simulink model "KR6_CLIK"  (R2018a)
settings: Solver=VariableStepAuto  StartTime=0.0  StopTime=inf  RelTol=1e-3
libraries: vrlib x8, KR6_Lib x1, realtime_pacer_lib x1
settings Model: Creator=Pedro Ramalho  LastModifiedBy=Pedro Ramalho

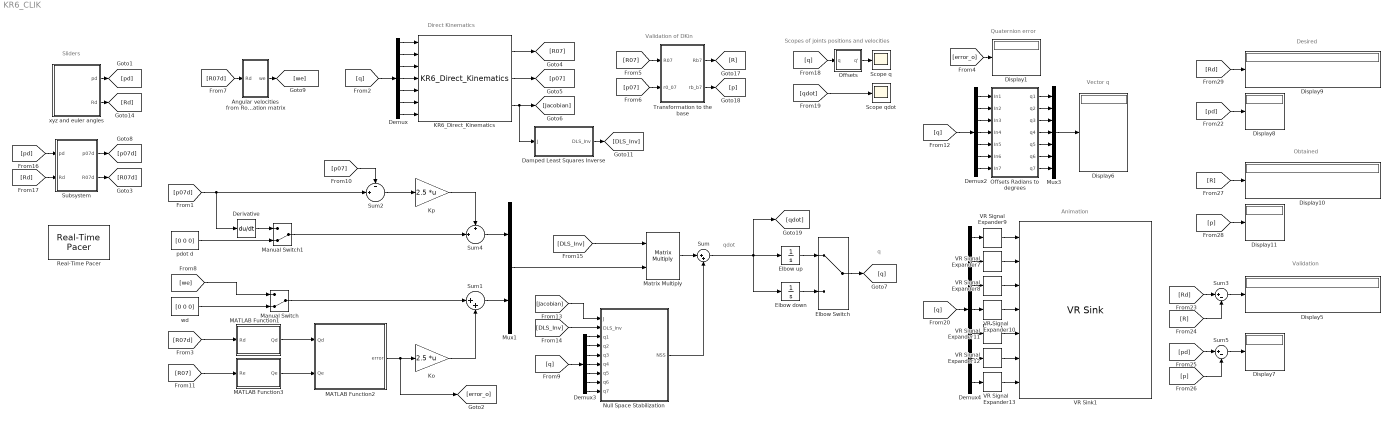
== system KR6_CLIK ==
  note: Direct Kinematics
  note: Validation of DKin
  note: qdot
  note: q
  note: Sliders
  note: Desired
  note: Obtained
  note: Validation
  note: Vector q
  note: Animation
  note: Scopes of joints positions and velocities
  note: Quaternion error
  Angular velocities from Rotation matrix : Subsystem
  Damped Least Squares Inverse : MATLAB Function  TreatAsAtomicUnit=on
  Demux{,2..4} (4 alike) : Demux  Outputs=7
  Derivative : Derivative
  Display{1,5..11} (8 alike) : Display
  Elbow Switch : ManualSwitch
  Elbow down : Integrator  InitialCondition=[0 0 0 -pi/2 0 0 pi]  ZeroCross=off
  Elbow up : Integrator  InitialCondition=[0 pi/8 -pi/2 0 0 0 pi]  ZeroCross=off
  KR6_Direct_Kinematics : KR6_Lib/KR6_Direct_Kinematics
  Ko : Gain  Gain=2.5  Multiplication=Matrix(K*u)
  Kp : Gain  Gain=2.5  Multiplication=Matrix(K*u)
  MATLAB Function1 : MATLAB Function  TreatAsAtomicUnit=on
  MATLAB Function2 : MATLAB Function  TreatAsAtomicUnit=on
  MATLAB Function3 : MATLAB Function  TreatAsAtomicUnit=on
  Manual Switch : ManualSwitch  CurrentSetting=0
  Manual Switch1 : ManualSwitch  CurrentSetting=0
  Matrix Multiply : Product  Multiplication=Matrix(*)
  Mux1 : Mux  Inputs=2
  Mux3 : Mux  Inputs=7
  Null Space Stabilization : MATLAB Function  TreatAsAtomicUnit=on
  Offsets : Subsystem
  Offsets Radians to degrees : Subsystem
  Real-Time Pacer : realtime_pacer_lib/Real-Time Pacer  simTimePerRealTime=1
  Scope q : Scope
  Scope qdot : Scope
  Subsystem : Subsystem
  Sum : Sum  Inputs=|++
  Sum1 : Sum  Inputs=|++
  Sum2 : Sum  Inputs=-|+||
  Sum3 : Sum  Inputs=|+-
  Sum4 : Sum  Inputs=+|+||
  Sum5 : Sum  Inputs=|+-
  Transformation to the base : Subsystem
  VR Signal Expander{7..8,10..13} (6 alike) : vrlib/VR Signal Expander  outwidth=4  outidx=4
      settings: SourceProductName=Simulink 3D Animation  SourceProductBaseCode=VR
  VR Signal Expander9 : vrlib/VR Signal Expander  outwidth=3  outidx=3
      settings: SourceProductName=Simulink 3D Animation  SourceProductBaseCode=VR
  VR Sink1 : vrlib/VR Sink  InstantiateOnLoad=on  SampleTime=0.1  ViewEnable=on  RemoteChange=off  RemoteView=off  FieldsWritten=Jt1_DH_dv.translation.3.1.1.double#Jt2_DH_dv.rotation.4.1.1.double#Jt3_DH_dv.rotation.4.1.1.double#Jt4_DH_dv.rotation.4.1.1.double#Jt5_DH_dv.rotation.4.1.1.double#Jt6_DH_dv.rotation.4.1.1.double#Jt7_DH_dv.rotation.4.1.1.double  WorldFileName=vrrobotKR6.wrl  WorldDescription=D-H Reference Frames for Virtual Reality Robot  AutoView=off  VideoDimensions=[]  AllowVariableSize=off
      settings: SourceProductBaseCode=VR
  pdot d : Constant  Value=[0 0 0]
  wd : Constant  Value=[0 0 0]
  xyz and euler angles : Subsystem  mask{px=0.20163, py=0.44482, pz=0.97382, phi=-75.4157, theta=-8.5121, psi=-120.3774}
      mask prompts: px "x"; py "y"; pz "z"
      mask DialogControl ParameterGroupVar_copy Prompt: Euler angles
  wires:
  KR6_Direct_Kinematics/1 -> [R07]
  KR6_Direct_Kinematics/2 -> [p07]
  KR6_Direct_Kinematics/3 -> [Jacobian], Damped Least Squares Inverse/1(J)
  Demux/1 -> KR6_Direct_Kinematics/1
  Demux/2 -> KR6_Direct_Kinematics/2
  Demux/3 -> KR6_Direct_Kinematics/3
  Demux/4 -> KR6_Direct_Kinematics/4
  Demux/5 -> KR6_Direct_Kinematics/5
  Demux/6 -> KR6_Direct_Kinematics/6
  Demux/7 -> KR6_Direct_Kinematics/7
  [q] -> Demux/1
  [p07d] -> Sum2/2, Derivative/1
  Transformation to the base/2(rb_b7) -> [p]
  [R07] -> Transformation to the base/1(R07)
  [p07] -> Transformation to the base/2(r0_07)
  [R07d] -> MATLAB Function1/1(Rd)
  MATLAB Function1/1(Qd) -> MATLAB Function2/1(Qd)
  MATLAB Function2/1(error) -> [error_o], Ko/1
  Ko/1 -> Sum1/2
  wd/1 -> Manual Switch/2
  Derivative/1 -> Manual Switch1/1
  pdot d/1 -> Manual Switch1/2
  [R07d] -> Angular velocities from Rotation matrix/1(Rd)
  Angular velocities from Rotation matrix/1(we) -> [we]
  [we] -> Manual Switch/1
  Manual Switch1/1 -> Sum4/2
  Kp/1 -> Sum4/1
  Manual Switch/1 -> Sum1/1
  Sum4/1 -> Mux1/1
  Sum1/1 -> Mux1/2
  Elbow up/1 -> Elbow Switch/1
  [p07] -> Sum2/1
  [R07] -> MATLAB Function3/1(Re)
  MATLAB Function3/1(Qe) -> MATLAB Function2/2(Qe)
  Offsets Radians to degrees/5(q5) -> Mux3/5
  Demux2/4 -> Offsets Radians to degrees/4(In4)
  Offsets Radians to degrees/3(q3) -> Mux3/3
  [q] -> Demux2/1
  Demux2/3 -> Offsets Radians to degrees/3(In3)
  Offsets Radians to degrees/1(q1) -> Mux3/1
  Demux2/6 -> Offsets Radians to degrees/6(In6)
  Demux2/5 -> Offsets Radians to degrees/5(In5)
  Offsets Radians to degrees/7(q7) -> Mux3/7
  Offsets Radians to degrees/4(q4) -> Mux3/4
  Mux3/1 -> Display6/1
  Offsets Radians to degrees/2(q2) -> Mux3/2
  Demux2/2 -> Offsets Radians to degrees/2(In2)
  Demux2/1 -> Offsets Radians to degrees/1(In1)
  Offsets Radians to degrees/6(q6) -> Mux3/6
  Demux2/7 -> Offsets Radians to degrees/7(In7)
  Damped Least Squares Inverse/1(DLS_Inv) -> [DLS_Inv]
  Matrix Multiply/1 -> Sum/1
  Null Space Stabilization/1(NSS) -> Sum/2
  Mux1/1 -> Matrix Multiply/2
  [q] -> Demux3/1
  Demux3/5 -> Null Space Stabilization/7(q5)
  Demux3/7 -> Null Space Stabilization/9(q7)
  Demux3/2 -> Null Space Stabilization/4(q2)
  Demux3/1 -> Null Space Stabilization/3(q1)
  Demux3/3 -> Null Space Stabilization/5(q3)
  Demux3/4 -> Null Space Stabilization/6(q4)
  Demux3/6 -> Null Space Stabilization/8(q6)
  [Jacobian] -> Null Space Stabilization/1(J)
  [DLS_Inv] -> Null Space Stabilization/2(DLS_Inv)
  [DLS_Inv] -> Matrix Multiply/1
  xyz and euler angles/2(Rd) -> [Rd]
  [pd] -> Subsystem/1(pd)
  [Rd] -> Subsystem/2(Rd)
  Subsystem/1(p07d) -> [p07d]
  xyz and euler angles/1(pd) -> [pd]
  Subsystem/2(R07d) -> [R07d]
  Sum5/1 -> Display7/1
  [Rd] -> Display9/1
  [R] -> Sum3/2
  Sum3/1 -> Display5/1
  [p] -> Sum5/2
  [Rd] -> Sum3/1
  [pd] -> Sum5/1
  [p] -> Display11/1
  [pd] -> Display8/1
  [R] -> Display10/1
  Offsets/1(q') -> Scope q/1
  [q] -> Offsets/1(q)
  Sum/1 -> Elbow down/1, Elbow up/1, [qdot]
  Elbow down/1 -> Elbow Switch/2
  Elbow Switch/1 -> [q]
  Sum2/1 -> Kp/1
  Transformation to the base/1(Rb7) -> [R]
  [qdot] -> Scope qdot/1
  Demux4/7 -> VR Signal Expander13/1
  Demux4/4 -> VR Signal Expander10/1
  Demux4/2 -> VR Signal Expander7/1
  Demux4/6 -> VR Signal Expander12/1
  Demux4/1 -> VR Signal Expander9/1
  [q] -> Demux4/1
  VR Signal Expander11/1 -> VR Sink1/5
  VR Signal Expander12/1 -> VR Sink1/6
  VR Signal Expander9/1 -> VR Sink1/1
  VR Signal Expander8/1 -> VR Sink1/3
  VR Signal Expander10/1 -> VR Sink1/4
  Demux4/5 -> VR Signal Expander11/1
  VR Signal Expander13/1 -> VR Sink1/7
  VR Signal Expander7/1 -> VR Sink1/2
  Demux4/3 -> VR Signal Expander8/1
  [error_o] -> Display1/1

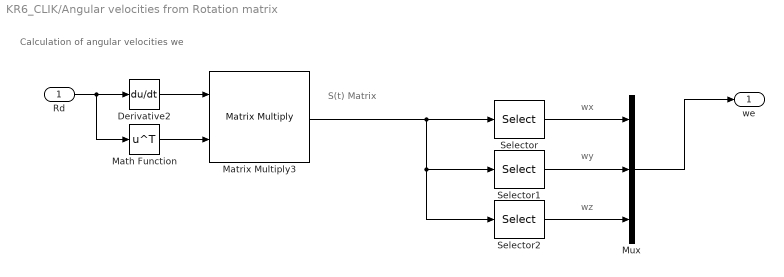
== system KR6_CLIK/Angular velocities from Rotation matrix ==
  note: S(t) Matrix
  note: wx
  note: Calculation of angular velocities we
  note: wz
  note: wy
  Rd : Inport
  Derivative2 : Derivative
  Math Function : Math  Operator=transpose  SaturateOnIntegerOverflow=on
  Matrix Multiply3 : Product  Multiplication=Matrix(*)
  Mux : Mux  Inputs=3
  Selector : Selector  NumberOfDimensions=2  InputPortWidth=3  IndexOptions=Index vector (dialog),Index vector (dialog)  Indices=[3],[2]  OutputSizes=1,1
  Selector1 : Selector  NumberOfDimensions=2  InputPortWidth=3  IndexOptions=Index vector (dialog),Index vector (dialog)  Indices=[1],[3]  OutputSizes=1,1
  Selector2 : Selector  NumberOfDimensions=2  InputPortWidth=3  IndexOptions=Index vector (dialog),Index vector (dialog)  Indices=[2],[1]  OutputSizes=1,1
  we : Outport
  wires:
  Mux/1 -> we/1
  Matrix Multiply3/1 -> Selector2/1, Selector1/1, Selector/1
  Rd/1 -> Math Function/1, Derivative2/1
  Derivative2/1 -> Matrix Multiply3/1
  Math Function/1 -> Matrix Multiply3/2
  Selector1/1 -> Mux/2
  Selector/1 -> Mux/1
  Selector2/1 -> Mux/3

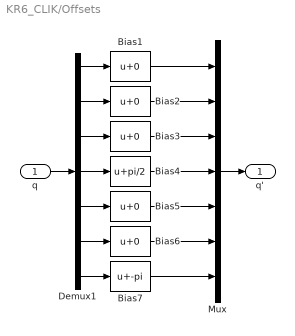
== system KR6_CLIK/Offsets ==
  q : Inport
  Bias{1..3,5..6} (5 alike) : Bias
  Bias4 : Bias  Bias=pi/2
  Bias7 : Bias  Bias=-pi
  Demux1 : Demux  Outputs=7
  Mux : Mux  Inputs=7
  q' : Outport
  wires:
  Bias2/1 -> Mux/2
  Bias3/1 -> Mux/3
  Bias4/1 -> Mux/4
  Bias5/1 -> Mux/5
  Bias6/1 -> Mux/6
  Bias7/1 -> Mux/7
  q/1 -> Demux1/1
  Demux1/1 -> Bias1/1
  Demux1/2 -> Bias2/1
  Demux1/3 -> Bias3/1
  Demux1/4 -> Bias4/1
  Demux1/5 -> Bias5/1
  Demux1/6 -> Bias6/1
  Demux1/7 -> Bias7/1
  Bias1/1 -> Mux/1
  Mux/1 -> q'/1

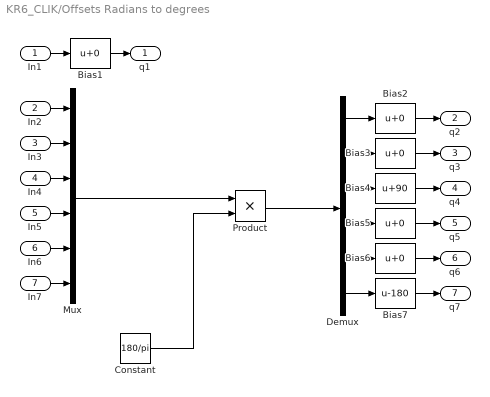
== system KR6_CLIK/Offsets Radians to degrees ==
  In1 : Inport
  In2 : Inport  Port=2
  In3 : Inport  Port=3
  In4 : Inport  Port=4
  In5 : Inport  Port=5
  In6 : Inport  Port=6
  In7 : Inport  Port=7
  Bias{1..3,5..6} (5 alike) : Bias
  Bias4 : Bias  Bias=90
  Bias7 : Bias  Bias=-180
  Constant : Constant  Value=180/pi
  Demux : Demux  Outputs=6
  Mux : Mux  Inputs=6
  Product : Product
  q1 : Outport
  q2 : Outport  Port=2
  q3 : Outport  Port=3
  q4 : Outport  Port=4
  q5 : Outport  Port=5
  q6 : Outport  Port=6
  q7 : Outport  Port=7
  wires:
  In1/1 -> Bias1/1
  Bias1/1 -> q1/1
  Mux/1 -> Product/1
  Constant/1 -> Product/2
  Product/1 -> Demux/1
  In2/1 -> Mux/1
  In3/1 -> Mux/2
  In4/1 -> Mux/3
  In5/1 -> Mux/4
  In6/1 -> Mux/5
  In7/1 -> Mux/6
  Demux/1 -> Bias2/1
  Demux/2 -> Bias3/1
  Demux/3 -> Bias4/1
  Demux/4 -> Bias5/1
  Demux/5 -> Bias6/1
  Demux/6 -> Bias7/1
  Bias2/1 -> q2/1
  Bias3/1 -> q3/1
  Bias4/1 -> q4/1
  Bias5/1 -> q5/1
  Bias6/1 -> q6/1
  Bias7/1 -> q7/1

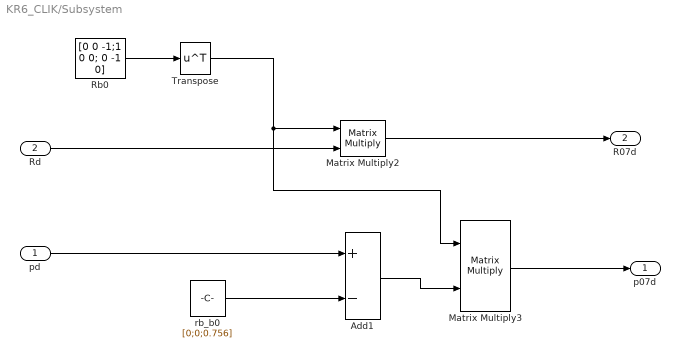
== system KR6_CLIK/Subsystem ==
  pd : Inport
  Rd : Inport  Port=2
  Add1 : Sum  Inputs=+-
  Matrix Multiply2 : Product  Multiplication=Matrix(*)
  Matrix Multiply3 : Product  Multiplication=Matrix(*)
  Rb0 : Constant  Value=[0 0 -1;1 0 0; 0 -1 0]
  Transpose : Math  Operator=transpose  SaturateOnIntegerOverflow=on
  rb_b0 : Constant  Value=[0;0;0.756]
  p07d : Outport
  R07d : Outport  Port=2
  wires:
  Add1/1 -> Matrix Multiply3/2
  Matrix Multiply3/1 -> p07d/1
  Rb0/1 -> Transpose/1
  Transpose/1 -> Matrix Multiply3/1, Matrix Multiply2/1
  Rd/1 -> Matrix Multiply2/2
  rb_b0/1 -> Add1/2
  pd/1 -> Add1/1
  Matrix Multiply2/1 -> R07d/1

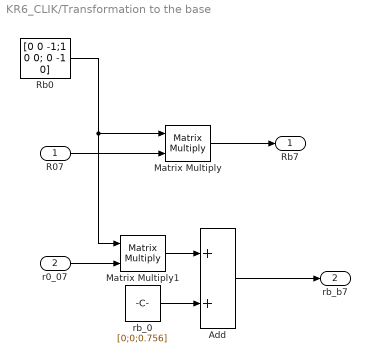
== system KR6_CLIK/Transformation to the base ==
  R07 : Inport
  r0_07 : Inport  Port=2
  Add : Sum
  Matrix Multiply : Product  Multiplication=Matrix(*)
  Matrix Multiply1 : Product  Multiplication=Matrix(*)
  Rb0 : Constant  Value=[0 0 -1;1 0 0; 0 -1 0]
  rb_0 : Constant  Value=[0;0;0.756]
  Rb7 : Outport
  rb_b7 : Outport  Port=2
  wires:
  Matrix Multiply1/1 -> Add/1
  R07/1 -> Matrix Multiply/2
  rb_0/1 -> Add/2
  Rb0/1 -> Matrix Multiply1/1, Matrix Multiply/1
  Matrix Multiply/1 -> Rb7/1
  r0_07/1 -> Matrix Multiply1/2
  Add/1 -> rb_b7/1

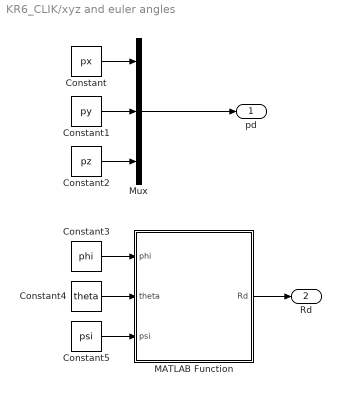
== system KR6_CLIK/xyz and euler angles ==
  Constant : Constant  Value=px
  Constant1 : Constant  Value=py
  Constant2 : Constant  Value=pz
  Constant3 : Constant  Value=phi
  Constant4 : Constant  Value=theta
  Constant5 : Constant  Value=psi
  MATLAB Function : MATLAB Function  TreatAsAtomicUnit=on
  Mux : Mux  Inputs=3
  pd : Outport
  Rd : Outport  Port=2
  wires:
  Constant/1 -> Mux/1
  Constant1/1 -> Mux/2
  Constant2/1 -> Mux/3
  Mux/1 -> pd/1
  Constant3/1 -> MATLAB Function/1(phi)
  Constant4/1 -> MATLAB Function/2(theta)
  Constant5/1 -> MATLAB Function/3(psi)
  MATLAB Function/1(Rd) -> Rd/1

== matlab function KR6_CLIK/MATLAB Function3 ==
  data: Re input; Qe output
function Qe = fcn(Re)


Qe=rotm2quat(Re);

== matlab function KR6_CLIK/xyz and euler angles/MATLAB Function ==
  data: phi input; Rd output; theta input; psi input
function Rd = fcn(phi,theta,psi)

eul = pi/180*[phi theta psi];
Rd = eul2rotm(eul);

end

== matlab function KR6_CLIK/Damped Least Squares Inverse ==
  data: J input size=[6 7]; DLS_Inv output
function DLS_Inv = fcn(J)
Jt = transpose(J);
k = 0.1;
%k = 0.1;
DLS_Inv = Jt/(J*Jt + k^2*eye(6));

== matlab function KR6_CLIK/MATLAB Function1 ==
  data: Rd input; Qd output
function Qd = fcn(Rd)


Qd=rotm2quat(Rd);

== matlab function KR6_CLIK/MATLAB Function2 ==
  data: Qd input; error output; Qe input
function error = ErrorComput(Qd, Qe)


error=Qe(1)*Qd(2:4)-Qd(1)*Qe(2:4)-cross(Qd(2:4),Qe(2:4));

== matlab function KR6_CLIK/Null Space Stabilization ==
  data: J input; DLS_Inv input; q1 input; NSS output; q2 input; q3 input; q4 input; q5 input; q6 input; q7 input
function NSS = fcn(J,DLS_Inv,q1,q2,q3,q4,q5,q6,q7)

qdot0 = [-(8100*q1)/(7*pi^2)/50;
     -(81*q2)/(2023*pi^2);
   -(2*q3 + pi)/(56*pi^2);
     -(81*q4)/(2023*pi^2);
    -(324*q5)/(9583*pi^2);
       -(9*q6)/(112*pi^2);
 -(2*q7 - 2*pi)/(56*pi^2)];

k0 = 0.01;
%k0 = 0.01;
NSS = (eye(7)- DLS_Inv * J)*qdot0*k0;
